simulink model "l4"  (R2012b)
settings: Solver=ode45  StartTime=0.0  StopTime=480  RelTol=1e-3
undefined symbols (not defined in the file): des, gcbh
settings Model: Creator=gick  LastModifiedBy=gick

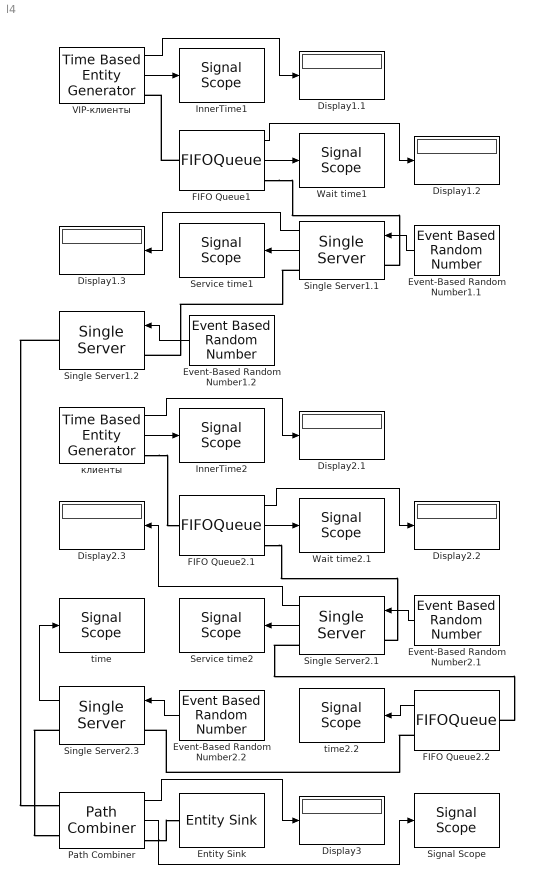
== system l4 ==
  Display1.1 : Display
  Display1.2 : Display
  Display1.3 : Display
  Display2.1 : Display
  Display2.2 : Display
  Display2.3 : Display
  Display3 : Display
  Entity Sink : EntitySink
  Event-Based Random Number1.1 : EventBasedRandomNumber  Distribution=Uniform  meanExp=15  minUnif=8  maxUnif=10  Seed=12
  Event-Based Random Number1.2 : EventBasedRandomNumber  meanExp=5  minUnif=3  maxUnif=3  Seed=12
  Event-Based Random Number2.1 : EventBasedRandomNumber  Distribution=Uniform  meanExp=15  minUnif=5  maxUnif=8  Seed=12
  Event-Based Random Number2.2 : EventBasedRandomNumber  meanExp=5  minUnif=3  maxUnif=3  Seed=12
  FIFO Queue1 : FIFOQueue  Capacity=20  StatNumberDeparted=on  StatAverageWait=on
      settings: OutputPortMap=o0,o2
  FIFO Queue2.1 : FIFOQueue  Capacity=20  StatNumberDeparted=on  StatAverageWait=on
      settings: OutputPortMap=o0,o2
  FIFO Queue2.2 : FIFOQueue  Capacity=20  StatAverageWait=on
      settings: OutputPortMap=o2
  InnerTime1 : SignalScope  LoadFcn=des.scope.CallbackSupport('seLoadFcn',gcbh)  StartFcn=des.scope.CallbackSupport('seStartFcn',gcbh)  StopFcn=des.scope.CallbackSupport('seStopFcn',gcbh)  ShowCountPlotted=on
      settings: CopyFcn=des.scope.CallbackSupport('seCopyFcn',gcbh)  DeleteFcn=des.scope.CallbackSupport('seDeleteFcn',gcbh)  PreSaveFcn=des.scope.CallbackSupport('sePreSaveFcn',gcbh)  NameChangeFcn=des.scope.CallbackSupport('seNameChangeFcn',gcbh)  OpenFcn=des.scope.CallbackSupport('seOpenFcn',gcbh)
  InnerTime2 : SignalScope  LoadFcn=des.scope.CallbackSupport('seLoadFcn',gcbh)  StartFcn=des.scope.CallbackSupport('seStartFcn',gcbh)  StopFcn=des.scope.CallbackSupport('seStopFcn',gcbh)  ShowCountPlotted=on
      settings: CopyFcn=des.scope.CallbackSupport('seCopyFcn',gcbh)  DeleteFcn=des.scope.CallbackSupport('seDeleteFcn',gcbh)  PreSaveFcn=des.scope.CallbackSupport('sePreSaveFcn',gcbh)  NameChangeFcn=des.scope.CallbackSupport('seNameChangeFcn',gcbh)  OpenFcn=des.scope.CallbackSupport('seOpenFcn',gcbh)
  Path Combiner : PathCombiner  NumberInputPorts=2  StatNumberDeparted=on  StatLastArrivalPort=on
      settings: OutputPortMap=o0,o1
  Service time1 : SignalScope  LoadFcn=des.scope.CallbackSupport('seLoadFcn',gcbh)  StartFcn=des.scope.CallbackSupport('seStartFcn',gcbh)  StopFcn=des.scope.CallbackSupport('seStopFcn',gcbh)  ShowCountPlotted=on
      settings: CopyFcn=des.scope.CallbackSupport('seCopyFcn',gcbh)  DeleteFcn=des.scope.CallbackSupport('seDeleteFcn',gcbh)  PreSaveFcn=des.scope.CallbackSupport('sePreSaveFcn',gcbh)  NameChangeFcn=des.scope.CallbackSupport('seNameChangeFcn',gcbh)  OpenFcn=des.scope.CallbackSupport('seOpenFcn',gcbh)
  Service time2 : SignalScope  LoadFcn=des.scope.CallbackSupport('seLoadFcn',gcbh)  StartFcn=des.scope.CallbackSupport('seStartFcn',gcbh)  StopFcn=des.scope.CallbackSupport('seStopFcn',gcbh)  ShowCountPlotted=on
      settings: CopyFcn=des.scope.CallbackSupport('seCopyFcn',gcbh)  DeleteFcn=des.scope.CallbackSupport('seDeleteFcn',gcbh)  PreSaveFcn=des.scope.CallbackSupport('sePreSaveFcn',gcbh)  NameChangeFcn=des.scope.CallbackSupport('seNameChangeFcn',gcbh)  OpenFcn=des.scope.CallbackSupport('seOpenFcn',gcbh)
  Signal Scope : SignalScope  LoadFcn=des.scope.CallbackSupport('seLoadFcn',gcbh)  StartFcn=des.scope.CallbackSupport('seStartFcn',gcbh)  StopFcn=des.scope.CallbackSupport('seStopFcn',gcbh)  ShowCountPlotted=on
      settings: CopyFcn=des.scope.CallbackSupport('seCopyFcn',gcbh)  DeleteFcn=des.scope.CallbackSupport('seDeleteFcn',gcbh)  PreSaveFcn=des.scope.CallbackSupport('sePreSaveFcn',gcbh)  NameChangeFcn=des.scope.CallbackSupport('seNameChangeFcn',gcbh)  OpenFcn=des.scope.CallbackSupport('seOpenFcn',gcbh)
  Single Server1.1 : SingleServer  ServiceTimeFrom=Signal port t  AttributeName=servtime  StatNumberDeparted=on  StatAverageWait=on
      settings: OutputPortMap=o0,o4
  Single Server1.2 : SingleServer  ServiceTimeFrom=Signal port t  AttributeName=servtime
  Single Server2.1 : SingleServer  ServiceTimeFrom=Signal port t  AttributeName=servtime  StatNumberDeparted=on  StatAverageWait=on
      settings: OutputPortMap=o0,o4
  Single Server2.3 : SingleServer  ServiceTimeFrom=Signal port t  AttributeName=servtime  StatAverageWait=on
      settings: OutputPortMap=o4
  VIP-клиенты : TimeBasedEntityGenerator  Distribution=Exponential  InitialSeed=12  Mean=20  StatNumberDeparted=on  StatAverageIntergenerationTime=on
      settings: OutputPortMap=o0,o2
  Wait time1 : SignalScope  LoadFcn=des.scope.CallbackSupport('seLoadFcn',gcbh)  StartFcn=des.scope.CallbackSupport('seStartFcn',gcbh)  StopFcn=des.scope.CallbackSupport('seStopFcn',gcbh)  ShowCountPlotted=on
      settings: CopyFcn=des.scope.CallbackSupport('seCopyFcn',gcbh)  DeleteFcn=des.scope.CallbackSupport('seDeleteFcn',gcbh)  PreSaveFcn=des.scope.CallbackSupport('sePreSaveFcn',gcbh)  NameChangeFcn=des.scope.CallbackSupport('seNameChangeFcn',gcbh)  OpenFcn=des.scope.CallbackSupport('seOpenFcn',gcbh)
  Wait time2.1 : SignalScope  LoadFcn=des.scope.CallbackSupport('seLoadFcn',gcbh)  StartFcn=des.scope.CallbackSupport('seStartFcn',gcbh)  StopFcn=des.scope.CallbackSupport('seStopFcn',gcbh)  ShowCountPlotted=on
      settings: CopyFcn=des.scope.CallbackSupport('seCopyFcn',gcbh)  DeleteFcn=des.scope.CallbackSupport('seDeleteFcn',gcbh)  PreSaveFcn=des.scope.CallbackSupport('sePreSaveFcn',gcbh)  NameChangeFcn=des.scope.CallbackSupport('seNameChangeFcn',gcbh)  OpenFcn=des.scope.CallbackSupport('seOpenFcn',gcbh)
  time : SignalScope  LoadFcn=des.scope.CallbackSupport('seLoadFcn',gcbh)  StartFcn=des.scope.CallbackSupport('seStartFcn',gcbh)  StopFcn=des.scope.CallbackSupport('seStopFcn',gcbh)  ShowCountPlotted=on
      settings: CopyFcn=des.scope.CallbackSupport('seCopyFcn',gcbh)  DeleteFcn=des.scope.CallbackSupport('seDeleteFcn',gcbh)  PreSaveFcn=des.scope.CallbackSupport('sePreSaveFcn',gcbh)  NameChangeFcn=des.scope.CallbackSupport('seNameChangeFcn',gcbh)  OpenFcn=des.scope.CallbackSupport('seOpenFcn',gcbh)
  time2.2 : SignalScope  LoadFcn=des.scope.CallbackSupport('seLoadFcn',gcbh)  StartFcn=des.scope.CallbackSupport('seStartFcn',gcbh)  StopFcn=des.scope.CallbackSupport('seStopFcn',gcbh)  ShowCountPlotted=on
      settings: CopyFcn=des.scope.CallbackSupport('seCopyFcn',gcbh)  DeleteFcn=des.scope.CallbackSupport('seDeleteFcn',gcbh)  PreSaveFcn=des.scope.CallbackSupport('sePreSaveFcn',gcbh)  NameChangeFcn=des.scope.CallbackSupport('seNameChangeFcn',gcbh)  OpenFcn=des.scope.CallbackSupport('seOpenFcn',gcbh)
  клиенты : TimeBasedEntityGenerator  Distribution=Exponential  InitialSeed=12  Mean=10  StatNumberDeparted=on  StatAverageIntergenerationTime=on
      settings: OutputPortMap=o0,o2
  wires:
  FIFO Queue2.1/2 -> Wait time2.1/1
  VIP-клиенты/1 -> Display1.1/1
  VIP-клиенты/2 -> InnerTime1/1
  FIFO Queue2.1/1 -> Display2.2/1
  Event-Based Random Number1.1/1 -> Single Server1.1/1
  Event-Based Random Number2.1/1 -> Single Server2.1/1
  Path Combiner/1 -> Display3/1
  клиенты/1 -> Display2.1/1
  клиенты/2 -> InnerTime2/1
  Path Combiner/2 -> Signal Scope/1
  Single Server1.1/1 -> Display1.3/1
  Single Server1.1/2 -> Service time1/1
  Single Server2.1/1 -> Display2.3/1
  Single Server2.1/2 -> Service time2/1
  FIFO Queue1/2 -> Wait time1/1
  FIFO Queue1/1 -> Display1.2/1
  Event-Based Random Number2.2/1 -> Single Server2.3/1
  FIFO Queue2.2/1 -> time2.2/1
  Single Server2.3/1 -> time/1
  Event-Based Random Number1.2/1 -> Single Server1.2/1
  connections:
  клиенты/RConn1 -- FIFO Queue2.1/LConn1
  FIFO Queue2.1/RConn1 -- Single Server2.1/LConn1
  Path Combiner/RConn1 -- Entity Sink/LConn1
  FIFO Queue1/LConn1 -- VIP-клиенты/RConn1
  FIFO Queue1/RConn1 -- Single Server1.1/LConn1
  Single Server2.1/RConn1 -- FIFO Queue2.2/LConn1
  FIFO Queue2.2/RConn1 -- Single Server2.3/LConn1
  Single Server2.3/RConn1 -- Path Combiner/LConn2
  Single Server1.1/RConn1 -- Single Server1.2/LConn1
  Single Server1.2/RConn1 -- Path Combiner/LConn1
